simulink model "upsampling"  (R2021a)
settings: Solver=VariableStepAuto  StartTime=0.0  StopTime=149  RelTol=1e-3
values from neighbouring files (symbols this model uses):
  n_sampling = 0.03    [datvis.m]
libraries: dspsrcs4 x12, simulink x1
settings Model: Creator=ASUS  LastModifiedBy=ASUS

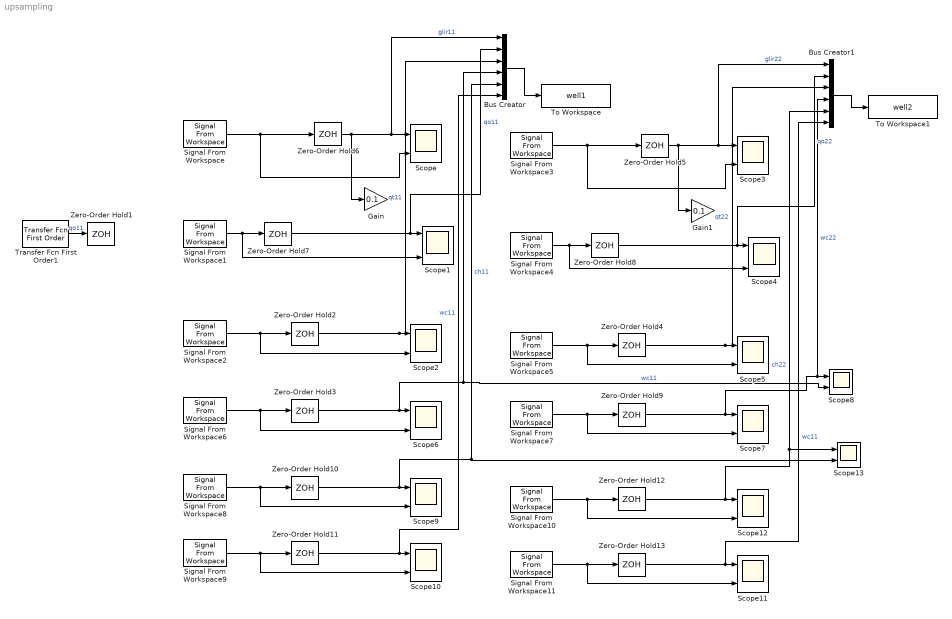
== system upsampling ==
  Bus Creator : BusCreator  Inputs=6
  Bus Creator1 : BusCreator  Inputs=6
  Gain : Gain  Gain=0.1
  Gain1 : Gain  Gain=0.1
  Scope{,2..3,5..13} (12 alike) : Scope  NumInputPorts=2
  Scope1 : Scope  NumInputPorts=3
  Scope4 : Scope  NumInputPorts=3
  Signal From Workspace : dspsrcs4/Signal From Workspace  X=glir1  Ts=1  nsamps=1  OutputAfterFinalValue=Setting to zero  ignoreOrWarnInputAndFrameLengths=off  OutputFrames=off
  Signal From Workspace1 : dspsrcs4/Signal From Workspace  X=qo1  Ts=1  nsamps=1  OutputAfterFinalValue=Setting to zero  ignoreOrWarnInputAndFrameLengths=off  OutputFrames=off
  Signal From Workspace10 : dspsrcs4/Signal From Workspace  X=ch2  Ts=1  nsamps=1  OutputAfterFinalValue=Setting to zero  ignoreOrWarnInputAndFrameLengths=off  OutputFrames=off
  Signal From Workspace11 : dspsrcs4/Signal From Workspace  X=gor2  Ts=1  nsamps=1  OutputAfterFinalValue=Setting to zero  ignoreOrWarnInputAndFrameLengths=off  OutputFrames=off
  Signal From Workspace2 : dspsrcs4/Signal From Workspace  X=qt1  Ts=1  nsamps=1  OutputAfterFinalValue=Setting to zero  ignoreOrWarnInputAndFrameLengths=off  OutputFrames=off
  Signal From Workspace3 : dspsrcs4/Signal From Workspace  X=glir2  Ts=1  nsamps=1  OutputAfterFinalValue=Setting to zero  ignoreOrWarnInputAndFrameLengths=off  OutputFrames=off
  Signal From Workspace4 : dspsrcs4/Signal From Workspace  X=qo2  Ts=1  nsamps=1  OutputAfterFinalValue=Setting to zero  ignoreOrWarnInputAndFrameLengths=off  OutputFrames=off
  Signal From Workspace5 : dspsrcs4/Signal From Workspace  X=qt2  Ts=1  nsamps=1  OutputAfterFinalValue=Setting to zero  ignoreOrWarnInputAndFrameLengths=off  OutputFrames=off
  Signal From Workspace6 : dspsrcs4/Signal From Workspace  X=wc1  Ts=1  nsamps=1  OutputAfterFinalValue=Setting to zero  ignoreOrWarnInputAndFrameLengths=off  OutputFrames=off
  Signal From Workspace7 : dspsrcs4/Signal From Workspace  X=wc2  Ts=1  nsamps=1  OutputAfterFinalValue=Setting to zero  ignoreOrWarnInputAndFrameLengths=off  OutputFrames=off
  Signal From Workspace8 : dspsrcs4/Signal From Workspace  X=ch1  Ts=1  nsamps=1  OutputAfterFinalValue=Setting to zero  ignoreOrWarnInputAndFrameLengths=off  OutputFrames=off
  Signal From Workspace9 : dspsrcs4/Signal From Workspace  X=gor1  Ts=1  nsamps=1  OutputAfterFinalValue=Setting to zero  ignoreOrWarnInputAndFrameLengths=off  OutputFrames=off
  To Workspace : ToWorkspace  VariableName=well1  SampleTime=n_sampling
      settings: Save2DSignal=2-D array (concatenate along first dimension)
  To Workspace1 : ToWorkspace  VariableName=well2  SampleTime=n_sampling
      settings: Save2DSignal=2-D array (concatenate along first dimension)
  Transfer Fcn First Order1 : simulink/Discrete/Transfer Fcn First Order  PoleZ=0.6456  ICPrevOutput=0.0  DoSatur=off
  Zero-Order Hold1 : ZeroOrderHold  SampleTime=n_sampling/2
  Zero-Order Hold{2..13} (12 alike) : ZeroOrderHold  SampleTime=n_sampling
  wires:
  Signal From Workspace/1 -> Zero-Order Hold6/1, Scope/2
  Bus Creator/1 -> To Workspace/1
  Zero-Order Hold2/1 -> Bus Creator/3, Scope2/1  "qt11"
  Zero-Order Hold6/1 -> Gain/1, Bus Creator/1, Scope/1  "glir11"
  Zero-Order Hold7/1 -> Bus Creator/2, Scope1/1  "qo11"
  Signal From Workspace1/1 -> Scope1/3, Zero-Order Hold7/1
  Signal From Workspace2/1 -> Zero-Order Hold2/1, Scope2/2
  Zero-Order Hold8/1 -> Bus Creator1/2, Scope4/1  "qo22"
  Zero-Order Hold5/1 -> Gain1/1, Bus Creator1/1, Scope3/1  "glir22"
  Signal From Workspace4/1 -> Scope4/3, Zero-Order Hold8/1
  Signal From Workspace5/1 -> Zero-Order Hold4/1, Scope5/2
  Bus Creator1/1 -> To Workspace1/1
  Zero-Order Hold4/1 -> Bus Creator1/3, Scope5/1  "qt22"
  Signal From Workspace3/1 -> Zero-Order Hold5/1, Scope3/2
  Signal From Workspace6/1 -> Zero-Order Hold3/1, Scope6/2
  Zero-Order Hold3/1 -> Scope8/2, Bus Creator/4, Scope6/1  "wc11"
  Zero-Order Hold9/1 -> Scope8/1, Bus Creator1/4, Scope7/1  "wc22"
  Signal From Workspace7/1 -> Zero-Order Hold9/1, Scope7/2
  Transfer Fcn First Order1/1 -> Zero-Order Hold1/1  "qo11"
  Zero-Order Hold10/1 -> Bus Creator/5, Scope13/2, Scope9/1  "ch11"
  Signal From Workspace8/1 -> Zero-Order Hold10/1, Scope9/2
  Zero-Order Hold11/1 -> Bus Creator/6, Scope10/1  "wc11"
  Signal From Workspace9/1 -> Zero-Order Hold11/1, Scope10/2
  Signal From Workspace11/1 -> Zero-Order Hold13/1, Scope11/2
  Zero-Order Hold13/1 -> Bus Creator1/6, Scope11/1  "wc11"
  Zero-Order Hold12/1 -> Scope13/1, Bus Creator1/5, Scope12/1  "ch22"
  Signal From Workspace10/1 -> Zero-Order Hold12/1, Scope12/2
